simulink model "cvd"  (R2024b)
settings: Solver=VariableStepAuto  StartTime=0.0  StopTime=40  RelTol=1e-3
undefined symbols (not defined in the file): Rcnv
libraries: cstblocks x1, simulink x1
settings Model: Creator=matth  LastModifiedBy=matth

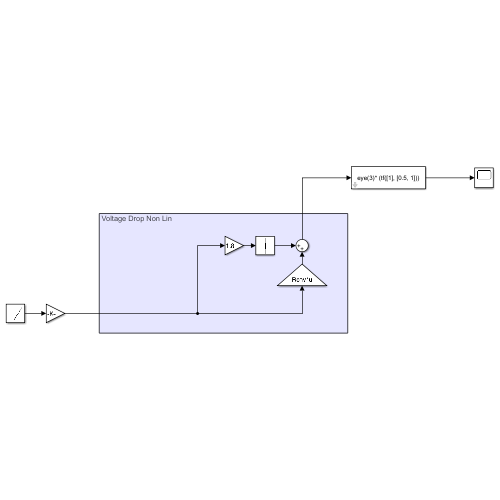
[thumbnail: Simulink's stored preview of the top-level diagram]
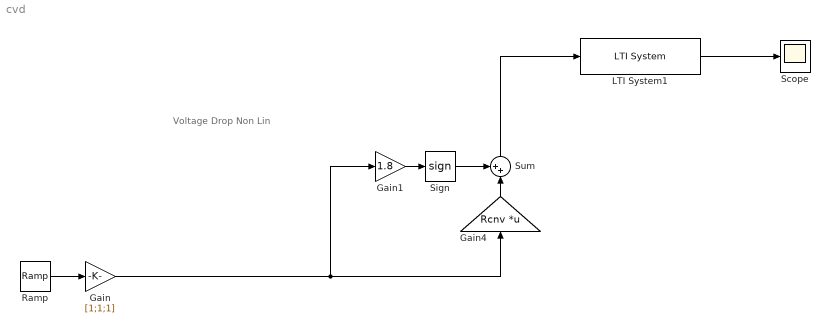
== system cvd ==
  note: Voltage Drop Non Lin
  Gain : Gain  Gain=[1;1;1]
  Gain1 : Gain  Gain=1.8
  Gain4 : Gain  Gain=Rcnv  Multiplication=Matrix(K*u)
  LTI System1 : cstblocks/LTI System  sys=eye(3)* (tf([1], [0.5, 1]))  IC=[]  PadeOrder=0
  Ramp : simulink/Sources/Ramp  slope=1  start=0  InitialOutput=-20
  Scope : Scope
  Sign : Signum
  Sum : Sum  Inputs=++|
  wires:
  Ramp/1 -> Gain/1
  Sum/1 -> LTI System1/1
  Gain1/1 -> Sign/1
  Gain/1 -> Gain4/1, Gain1/1
  Gain4/1 -> Sum/2
  Sign/1 -> Sum/1
  LTI System1/1 -> Scope/1
